simulink model "TST_StSys_StrtCtl"  (R2016b)
settings: Solver=FixedStepDiscrete  StartTime=0.0  StopTime=simTime  FixedStep=sampleTime  RelTol=1e-3
values from neighbouring files (symbols this model uses):
  testCase = 1    [initTST_StSys_StrtCtl_001.m]    (also in initTST_StSys_StrtCtl_002.m = 2)
libraries: simulink x5, UnitTest_Lib x2
settings Model: Creator=xuxingpei  LastModifiedBy=xuxingpei
settings DebuggingCC: SignalRangeChecking=error

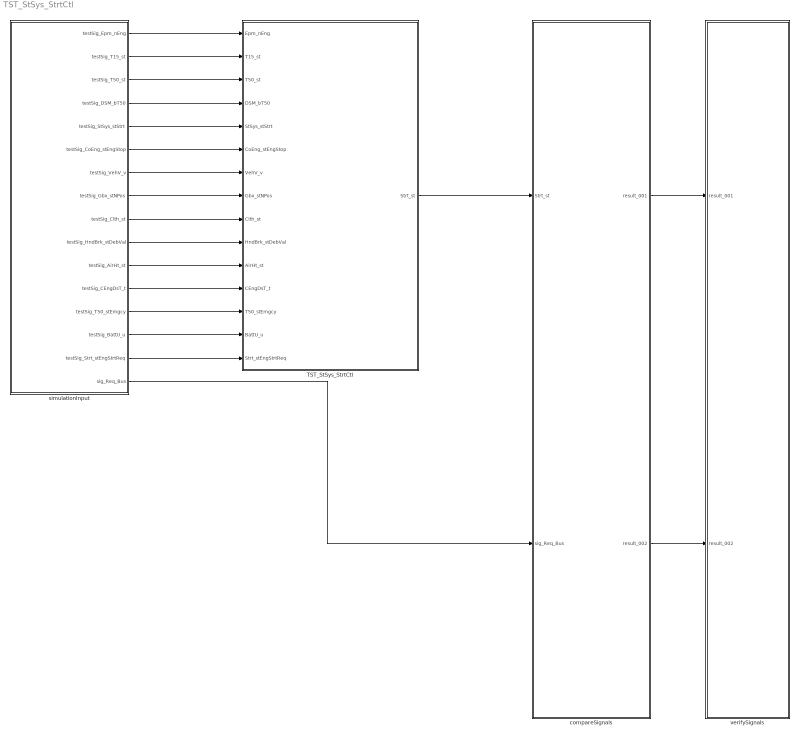
== system TST_StSys_StrtCtl ==
  TST_StSys_StrtCtl : Subsystem
  compareSignals : Subsystem
  simulationInput : Subsystem
  verifySignals : Subsystem
  wires:
  simulationInput/1(testSig_Epm_nEng) -> TST_StSys_StrtCtl/1(Epm_nEng)
  simulationInput/2(testSig_T15_st) -> TST_StSys_StrtCtl/2(T15_st)
  simulationInput/3(testSig_T50_st) -> TST_StSys_StrtCtl/3(T50_st)
  simulationInput/4(testSig_DSM_bT50) -> TST_StSys_StrtCtl/4(DSM_bT50)
  simulationInput/5(testSig_StSys_stStrt) -> TST_StSys_StrtCtl/5(StSys_stStrt)
  simulationInput/6(testSig_CoEng_stEngStop) -> TST_StSys_StrtCtl/6(CoEng_stEngStop)
  simulationInput/7(testSig_VehV_v) -> TST_StSys_StrtCtl/7(VehV_v)
  simulationInput/8(testSig_Gbx_stNPos) -> TST_StSys_StrtCtl/8(Gbx_stNPos)
  simulationInput/9(testSig_Clth_st) -> TST_StSys_StrtCtl/9(Clth_st)
  simulationInput/10(testSig_HndBrk_stDebVal) -> TST_StSys_StrtCtl/10(HndBrk_stDebVal)
  simulationInput/11(testSig_AirHt_st) -> TST_StSys_StrtCtl/11(AirHt_st)
  simulationInput/12(testSig_CEngDsT_t) -> TST_StSys_StrtCtl/12(CEngDsT_t)
  simulationInput/13(testSig_T50_stEmgcy) -> TST_StSys_StrtCtl/13(T50_stEmgcy)
  simulationInput/14(testSig_BattU_u) -> TST_StSys_StrtCtl/14(BattU_u)
  simulationInput/15(testSig_Strt_stEngStrtReq) -> TST_StSys_StrtCtl/15(Strt_stEngStrtReq)
  TST_StSys_StrtCtl/1(Strt_st) -> compareSignals/1(Strt_st)
  simulationInput/16(sig_Req_Bus) -> compareSignals/2(sig_Req_Bus)
  compareSignals/1(result_001) -> verifySignals/1(result_001)
  compareSignals/2(result_002) -> verifySignals/2(result_002)

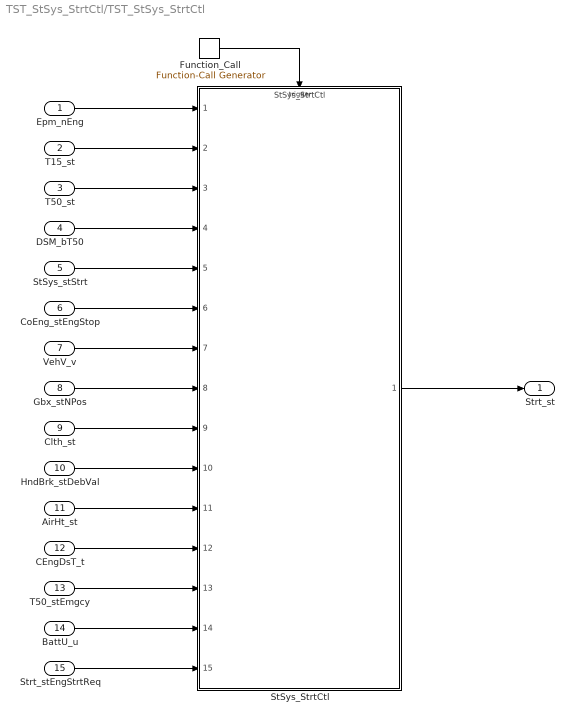
== system TST_StSys_StrtCtl/TST_StSys_StrtCtl ==
  Epm_nEng : Inport
  T15_st : Inport  Port=2
  T50_st : Inport  Port=3
  DSM_bT50 : Inport  Port=4
  StSys_stStrt : Inport  Port=5
  CoEng_stEngStop : Inport  Port=6
  VehV_v : Inport  Port=7
  Gbx_stNPos : Inport  Port=8
  Clth_st : Inport  Port=9
  HndBrk_stDebVal : Inport  Port=10
  AirHt_st : Inport  Port=11
  CEngDsT_t : Inport  Port=12
  T50_stEmgcy : Inport  Port=13
  BattU_u : Inport  Port=14
  Strt_stEngStrtReq : Inport  Port=15
  Function_Call : simulink/Ports & Subsystems/Function-Call Generator  sample_time=sampleTime  numberOfIterations=1
  StSys_StrtCtl : ModelReference  ModelNameDialog=StSys_StrtCtl  SimulationMode=Normal  ModelReferenceVersion=1.583  TriggerPortName=function  TriggerPortTriggerType=function-call  TriggerPortStatesWhenEnabling=held
  Strt_st : Outport
  wires:
  Function_Call/1 -> StSys_StrtCtl/Trigger
  Epm_nEng/1 -> StSys_StrtCtl/1
  T15_st/1 -> StSys_StrtCtl/2
  T50_st/1 -> StSys_StrtCtl/3
  DSM_bT50/1 -> StSys_StrtCtl/4
  StSys_stStrt/1 -> StSys_StrtCtl/5
  CoEng_stEngStop/1 -> StSys_StrtCtl/6
  VehV_v/1 -> StSys_StrtCtl/7
  Gbx_stNPos/1 -> StSys_StrtCtl/8
  Clth_st/1 -> StSys_StrtCtl/9
  HndBrk_stDebVal/1 -> StSys_StrtCtl/10
  AirHt_st/1 -> StSys_StrtCtl/11
  CEngDsT_t/1 -> StSys_StrtCtl/12
  T50_stEmgcy/1 -> StSys_StrtCtl/13
  BattU_u/1 -> StSys_StrtCtl/14
  Strt_stEngStrtReq/1 -> StSys_StrtCtl/15
  StSys_StrtCtl/1 -> Strt_st/1

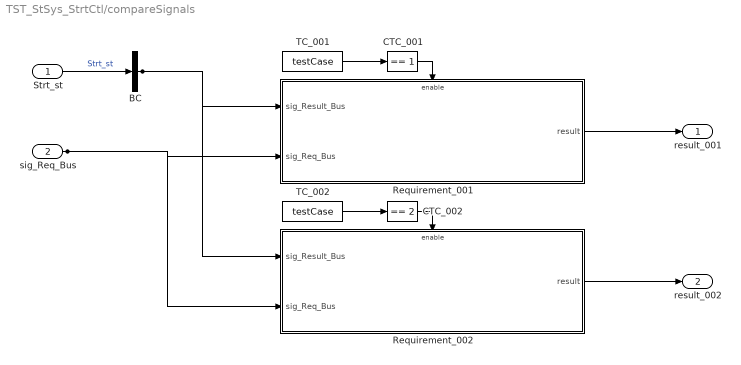
== system TST_StSys_StrtCtl/compareSignals ==
  Strt_st : Inport
  sig_Req_Bus : Inport  Port=2
  BC : BusCreator  Inputs=1
  CTC_001 : simulink/Logic and Bit Operations/Compare To Constant  relop===  const=1  OutDataTypeStr=boolean
  CTC_002 : simulink/Logic and Bit Operations/Compare To Constant  relop===  const=2  OutDataTypeStr=boolean
  Requirement_001 : Subsystem
  Requirement_002 : Subsystem
  TC_001 : Constant  Value=testCase
  TC_002 : Constant  Value=testCase
  result_001 : Outport
  result_002 : Outport  Port=2
  wires:
  Strt_st/1 -> BC/1  "Strt_st"
  TC_001/1 -> CTC_001/1
  CTC_001/1 -> Requirement_001/Enable
  sig_Req_Bus/1 -> Requirement_001/2(sig_Req_Bus), Requirement_002/2(sig_Req_Bus)
  BC/1 -> Requirement_001/1(sig_Result_Bus), Requirement_002/1(sig_Result_Bus)
  Requirement_001/1(result) -> result_001/1
  TC_002/1 -> CTC_002/1
  CTC_002/1 -> Requirement_002/Enable
  Requirement_002/1(result) -> result_002/1

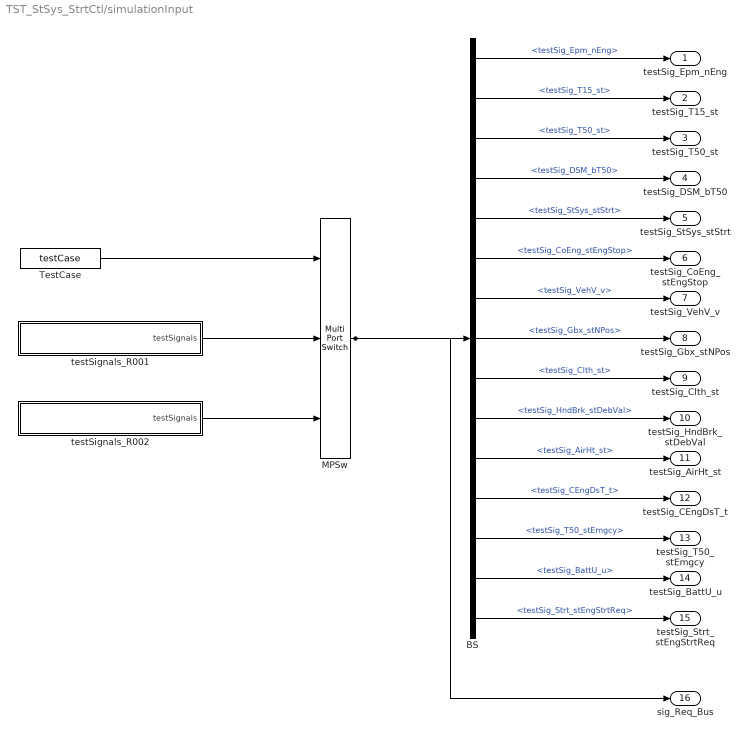
== system TST_StSys_StrtCtl/simulationInput ==
  BS : BusSelector  OutputSignals=testSig_Epm_nEng,testSig_T15_st,testSig_T50_st,testSig_DSM_bT50,testSig_StSys_stStrt,testSig_CoEng_stEngStop,testSig_VehV_v,testSig_Gbx_stNPos,testSig_Clth_st,testSig_HndBrk_stDebVal,testSig_AirHt_st,testSig_CEngDsT_t,testSig_T50_stEmgcy,testSig_BattU_u,testSig_Strt_stEngStrtReq
  MPSw : MultiPortSwitch  Inputs=2  SaturateOnIntegerOverflow=on  InputSameDT=on
  TestCase : Constant  Value=testCase
  testSignals_R001 : Subsystem
  testSignals_R002 : Subsystem
  testSig_Epm_nEng : Outport
  testSig_T15_st : Outport  Port=2
  testSig_T50_st : Outport  Port=3
  testSig_DSM_bT50 : Outport  Port=4
  testSig_StSys_stStrt : Outport  Port=5
  testSig_CoEng_stEngStop : Outport  Port=6
  testSig_VehV_v : Outport  Port=7
  testSig_Gbx_stNPos : Outport  Port=8
  testSig_Clth_st : Outport  Port=9
  testSig_HndBrk_stDebVal : Outport  Port=10
  testSig_AirHt_st : Outport  Port=11
  testSig_CEngDsT_t : Outport  Port=12
  testSig_T50_stEmgcy : Outport  Port=13
  testSig_BattU_u : Outport  Port=14
  testSig_Strt_stEngStrtReq : Outport  Port=15
  sig_Req_Bus : Outport  Port=16
  wires:
  BS/1 -> testSig_Epm_nEng/1  "<testSig_Epm_nEng>"
  BS/2 -> testSig_T15_st/1  "<testSig_T15_st>"
  BS/3 -> testSig_T50_st/1  "<testSig_T50_st>"
  BS/4 -> testSig_DSM_bT50/1  "<testSig_DSM_bT50>"
  BS/5 -> testSig_StSys_stStrt/1  "<testSig_StSys_stStrt>"
  BS/6 -> testSig_CoEng_stEngStop/1  "<testSig_CoEng_stEngStop>"
  BS/7 -> testSig_VehV_v/1  "<testSig_VehV_v>"
  BS/8 -> testSig_Gbx_stNPos/1  "<testSig_Gbx_stNPos>"
  BS/9 -> testSig_Clth_st/1  "<testSig_Clth_st>"
  BS/10 -> testSig_HndBrk_stDebVal/1  "<testSig_HndBrk_stDebVal>"
  BS/11 -> testSig_AirHt_st/1  "<testSig_AirHt_st>"
  BS/12 -> testSig_CEngDsT_t/1  "<testSig_CEngDsT_t>"
  BS/13 -> testSig_T50_stEmgcy/1  "<testSig_T50_stEmgcy>"
  BS/14 -> testSig_BattU_u/1  "<testSig_BattU_u>"
  BS/15 -> testSig_Strt_stEngStrtReq/1  "<testSig_Strt_stEngStrtReq>"
  MPSw/1 -> BS/1, sig_Req_Bus/1
  TestCase/1 -> MPSw/1
  testSignals_R001/1(testSignals) -> MPSw/2
  testSignals_R002/1(testSignals) -> MPSw/3

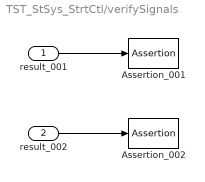
== system TST_StSys_StrtCtl/verifySignals ==
  result_001 : Inport
  result_002 : Inport  Port=2
  Assertion_001 : Assertion  Enabled=off
  Assertion_002 : Assertion  Enabled=off
  wires:
  result_001/1 -> Assertion_001/1
  result_002/1 -> Assertion_002/1

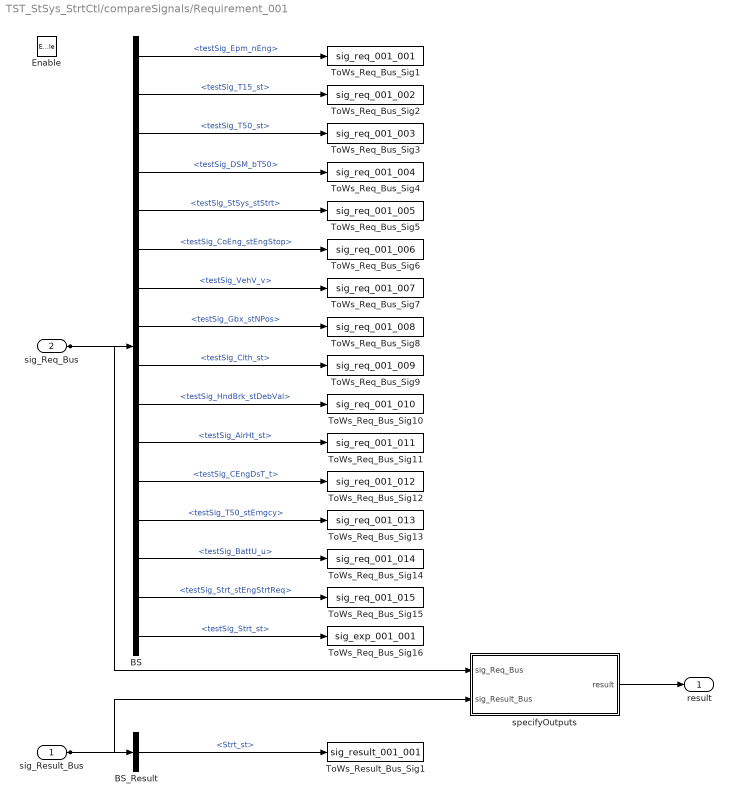
== system TST_StSys_StrtCtl/compareSignals/Requirement_001 ==
  sig_Result_Bus : Inport
  sig_Req_Bus : Inport  Port=2
  Enable : EnablePort
  BS : BusSelector  OutputSignals=testSig_Epm_nEng,testSig_T15_st,testSig_T50_st,testSig_DSM_bT50,testSig_StSys_stStrt,testSig_CoEng_stEngStop,testSig_VehV_v,testSig_Gbx_stNPos,testSig_Clth_st,testSig_HndBrk_stDebVal,testSig_AirHt_st,testSig_CEngDsT_t,testSig_T50_stEmgcy,testSig_BattU_u,testSig_Strt_stEngStrtReq,testSig_Strt_st
  BS_Result : BusSelector  OutputSignals=Strt_st
  ToWs_Req_Bus_Sig1 : ToWorkspace  VariableName=sig_req_001_001  SaveFormat=Structure With Time
  ToWs_Req_Bus_Sig10 : ToWorkspace  VariableName=sig_req_001_010  SaveFormat=Structure With Time
  ToWs_Req_Bus_Sig11 : ToWorkspace  VariableName=sig_req_001_011  SaveFormat=Structure With Time
  ToWs_Req_Bus_Sig12 : ToWorkspace  VariableName=sig_req_001_012  SaveFormat=Structure With Time
  ToWs_Req_Bus_Sig13 : ToWorkspace  VariableName=sig_req_001_013  SaveFormat=Structure With Time
  ToWs_Req_Bus_Sig14 : ToWorkspace  VariableName=sig_req_001_014  SaveFormat=Structure With Time
  ToWs_Req_Bus_Sig15 : ToWorkspace  VariableName=sig_req_001_015  SaveFormat=Structure With Time
  ToWs_Req_Bus_Sig16 : ToWorkspace  VariableName=sig_exp_001_001  SaveFormat=Structure With Time
  ToWs_Req_Bus_Sig2 : ToWorkspace  VariableName=sig_req_001_002  SaveFormat=Structure With Time
  ToWs_Req_Bus_Sig3 : ToWorkspace  VariableName=sig_req_001_003  SaveFormat=Structure With Time
  ToWs_Req_Bus_Sig4 : ToWorkspace  VariableName=sig_req_001_004  SaveFormat=Structure With Time
  ToWs_Req_Bus_Sig5 : ToWorkspace  VariableName=sig_req_001_005  SaveFormat=Structure With Time
  ToWs_Req_Bus_Sig6 : ToWorkspace  VariableName=sig_req_001_006  SaveFormat=Structure With Time
  ToWs_Req_Bus_Sig7 : ToWorkspace  VariableName=sig_req_001_007  SaveFormat=Structure With Time
  ToWs_Req_Bus_Sig8 : ToWorkspace  VariableName=sig_req_001_008  SaveFormat=Structure With Time
  ToWs_Req_Bus_Sig9 : ToWorkspace  VariableName=sig_req_001_009  SaveFormat=Structure With Time
  ToWs_Result_Bus_Sig1 : ToWorkspace  VariableName=sig_result_001_001  SaveFormat=Structure With Time
  specifyOutputs : Subsystem
  result : Outport
  wires:
  sig_Req_Bus/1 -> BS/1, specifyOutputs/1(sig_Req_Bus)
  BS/1 -> ToWs_Req_Bus_Sig1/1  "<testSig_Epm_nEng>"
  BS/2 -> ToWs_Req_Bus_Sig2/1  "<testSig_T15_st>"
  BS/3 -> ToWs_Req_Bus_Sig3/1  "<testSig_T50_st>"
  BS/4 -> ToWs_Req_Bus_Sig4/1  "<testSig_DSM_bT50>"
  BS/5 -> ToWs_Req_Bus_Sig5/1  "<testSig_StSys_stStrt>"
  BS/6 -> ToWs_Req_Bus_Sig6/1  "<testSig_CoEng_stEngStop>"
  BS/7 -> ToWs_Req_Bus_Sig7/1  "<testSig_VehV_v>"
  BS/8 -> ToWs_Req_Bus_Sig8/1  "<testSig_Gbx_stNPos>"
  BS/9 -> ToWs_Req_Bus_Sig9/1  "<testSig_Clth_st>"
  BS/10 -> ToWs_Req_Bus_Sig10/1  "<testSig_HndBrk_stDebVal>"
  BS/11 -> ToWs_Req_Bus_Sig11/1  "<testSig_AirHt_st>"
  BS/12 -> ToWs_Req_Bus_Sig12/1  "<testSig_CEngDsT_t>"
  BS/13 -> ToWs_Req_Bus_Sig13/1  "<testSig_T50_stEmgcy>"
  BS/14 -> ToWs_Req_Bus_Sig14/1  "<testSig_BattU_u>"
  BS/15 -> ToWs_Req_Bus_Sig15/1  "<testSig_Strt_stEngStrtReq>"
  BS/16 -> ToWs_Req_Bus_Sig16/1  "<testSig_Strt_st>"
  sig_Result_Bus/1 -> BS_Result/1, specifyOutputs/2(sig_Result_Bus)
  BS_Result/1 -> ToWs_Result_Bus_Sig1/1  "<Strt_st>"
  specifyOutputs/1(result) -> result/1

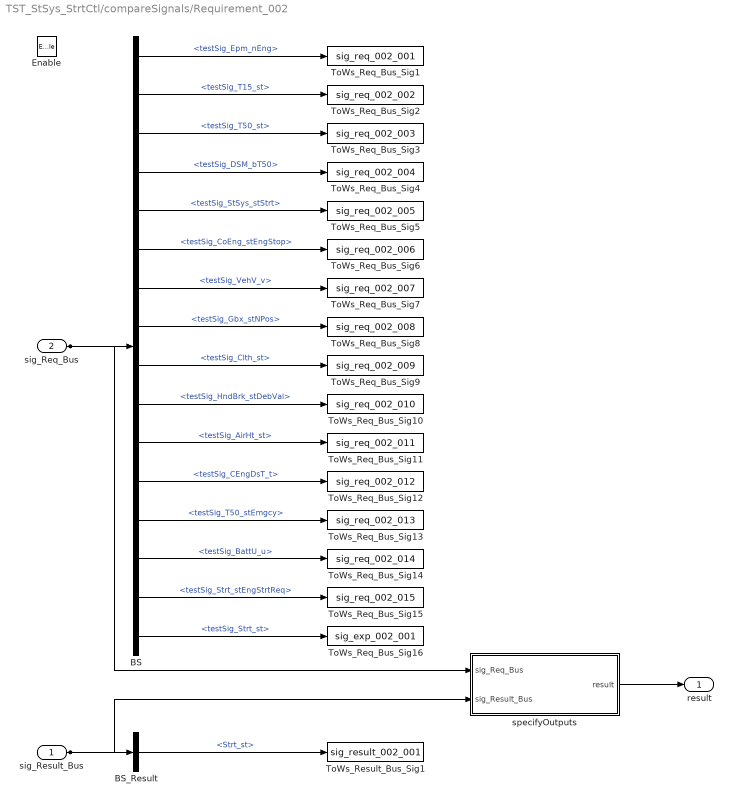
== system TST_StSys_StrtCtl/compareSignals/Requirement_002 ==
  sig_Result_Bus : Inport
  sig_Req_Bus : Inport  Port=2
  Enable : EnablePort
  BS : BusSelector  OutputSignals=testSig_Epm_nEng,testSig_T15_st,testSig_T50_st,testSig_DSM_bT50,testSig_StSys_stStrt,testSig_CoEng_stEngStop,testSig_VehV_v,testSig_Gbx_stNPos,testSig_Clth_st,testSig_HndBrk_stDebVal,testSig_AirHt_st,testSig_CEngDsT_t,testSig_T50_stEmgcy,testSig_BattU_u,testSig_Strt_stEngStrtReq,testSig_Strt_st
  BS_Result : BusSelector  OutputSignals=Strt_st
  ToWs_Req_Bus_Sig1 : ToWorkspace  VariableName=sig_req_002_001  SaveFormat=Structure With Time
  ToWs_Req_Bus_Sig10 : ToWorkspace  VariableName=sig_req_002_010  SaveFormat=Structure With Time
  ToWs_Req_Bus_Sig11 : ToWorkspace  VariableName=sig_req_002_011  SaveFormat=Structure With Time
  ToWs_Req_Bus_Sig12 : ToWorkspace  VariableName=sig_req_002_012  SaveFormat=Structure With Time
  ToWs_Req_Bus_Sig13 : ToWorkspace  VariableName=sig_req_002_013  SaveFormat=Structure With Time
  ToWs_Req_Bus_Sig14 : ToWorkspace  VariableName=sig_req_002_014  SaveFormat=Structure With Time
  ToWs_Req_Bus_Sig15 : ToWorkspace  VariableName=sig_req_002_015  SaveFormat=Structure With Time
  ToWs_Req_Bus_Sig16 : ToWorkspace  VariableName=sig_exp_002_001  SaveFormat=Structure With Time
  ToWs_Req_Bus_Sig2 : ToWorkspace  VariableName=sig_req_002_002  SaveFormat=Structure With Time
  ToWs_Req_Bus_Sig3 : ToWorkspace  VariableName=sig_req_002_003  SaveFormat=Structure With Time
  ToWs_Req_Bus_Sig4 : ToWorkspace  VariableName=sig_req_002_004  SaveFormat=Structure With Time
  ToWs_Req_Bus_Sig5 : ToWorkspace  VariableName=sig_req_002_005  SaveFormat=Structure With Time
  ToWs_Req_Bus_Sig6 : ToWorkspace  VariableName=sig_req_002_006  SaveFormat=Structure With Time
  ToWs_Req_Bus_Sig7 : ToWorkspace  VariableName=sig_req_002_007  SaveFormat=Structure With Time
  ToWs_Req_Bus_Sig8 : ToWorkspace  VariableName=sig_req_002_008  SaveFormat=Structure With Time
  ToWs_Req_Bus_Sig9 : ToWorkspace  VariableName=sig_req_002_009  SaveFormat=Structure With Time
  ToWs_Result_Bus_Sig1 : ToWorkspace  VariableName=sig_result_002_001  SaveFormat=Structure With Time
  specifyOutputs : Subsystem
  result : Outport
  wires:
  sig_Req_Bus/1 -> BS/1, specifyOutputs/1(sig_Req_Bus)
  BS/1 -> ToWs_Req_Bus_Sig1/1  "<testSig_Epm_nEng>"
  BS/2 -> ToWs_Req_Bus_Sig2/1  "<testSig_T15_st>"
  BS/3 -> ToWs_Req_Bus_Sig3/1  "<testSig_T50_st>"
  BS/4 -> ToWs_Req_Bus_Sig4/1  "<testSig_DSM_bT50>"
  BS/5 -> ToWs_Req_Bus_Sig5/1  "<testSig_StSys_stStrt>"
  BS/6 -> ToWs_Req_Bus_Sig6/1  "<testSig_CoEng_stEngStop>"
  BS/7 -> ToWs_Req_Bus_Sig7/1  "<testSig_VehV_v>"
  BS/8 -> ToWs_Req_Bus_Sig8/1  "<testSig_Gbx_stNPos>"
  BS/9 -> ToWs_Req_Bus_Sig9/1  "<testSig_Clth_st>"
  BS/10 -> ToWs_Req_Bus_Sig10/1  "<testSig_HndBrk_stDebVal>"
  BS/11 -> ToWs_Req_Bus_Sig11/1  "<testSig_AirHt_st>"
  BS/12 -> ToWs_Req_Bus_Sig12/1  "<testSig_CEngDsT_t>"
  BS/13 -> ToWs_Req_Bus_Sig13/1  "<testSig_T50_stEmgcy>"
  BS/14 -> ToWs_Req_Bus_Sig14/1  "<testSig_BattU_u>"
  BS/15 -> ToWs_Req_Bus_Sig15/1  "<testSig_Strt_stEngStrtReq>"
  BS/16 -> ToWs_Req_Bus_Sig16/1  "<testSig_Strt_st>"
  sig_Result_Bus/1 -> BS_Result/1, specifyOutputs/2(sig_Result_Bus)
  BS_Result/1 -> ToWs_Result_Bus_Sig1/1  "<Strt_st>"
  specifyOutputs/1(result) -> result/1

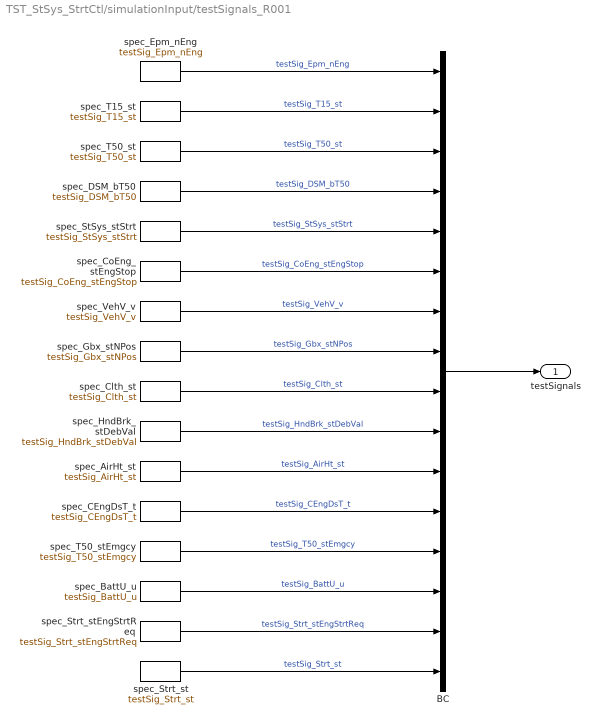
== system TST_StSys_StrtCtl/simulationInput/testSignals_R001 ==
  BC : BusCreator  Inputs=16
  spec_AirHt_st : FromWorkspace  VariableName=testSig_AirHt_st  Interpolate=off  OutputAfterFinalValue=Holding final value
  spec_BattU_u : FromWorkspace  VariableName=testSig_BattU_u  Interpolate=off  OutputAfterFinalValue=Holding final value
  spec_CEngDsT_t : FromWorkspace  VariableName=testSig_CEngDsT_t  Interpolate=off  OutputAfterFinalValue=Holding final value
  spec_Clth_st : FromWorkspace  VariableName=testSig_Clth_st  Interpolate=off  OutputAfterFinalValue=Holding final value
  spec_CoEng_stEngStop : FromWorkspace  VariableName=testSig_CoEng_stEngStop  Interpolate=off  OutputAfterFinalValue=Holding final value
  spec_DSM_bT50 : FromWorkspace  VariableName=testSig_DSM_bT50  Interpolate=off  OutputAfterFinalValue=Holding final value
  spec_Epm_nEng : FromWorkspace  VariableName=testSig_Epm_nEng  Interpolate=off  OutputAfterFinalValue=Holding final value
  spec_Gbx_stNPos : FromWorkspace  VariableName=testSig_Gbx_stNPos  Interpolate=off  OutputAfterFinalValue=Holding final value
  spec_HndBrk_stDebVal : FromWorkspace  VariableName=testSig_HndBrk_stDebVal  Interpolate=off  OutputAfterFinalValue=Holding final value
  spec_StSys_stStrt : FromWorkspace  VariableName=testSig_StSys_stStrt  Interpolate=off  OutputAfterFinalValue=Holding final value
  spec_Strt_st : FromWorkspace  VariableName=testSig_Strt_st  Interpolate=off  OutputAfterFinalValue=Holding final value
  spec_Strt_stEngStrtReq : FromWorkspace  VariableName=testSig_Strt_stEngStrtReq  Interpolate=off  OutputAfterFinalValue=Holding final value
  spec_T15_st : FromWorkspace  VariableName=testSig_T15_st  Interpolate=off  OutputAfterFinalValue=Holding final value
  spec_T50_st : FromWorkspace  VariableName=testSig_T50_st  Interpolate=off  OutputAfterFinalValue=Holding final value
  spec_T50_stEmgcy : FromWorkspace  VariableName=testSig_T50_stEmgcy  Interpolate=off  OutputAfterFinalValue=Holding final value
  spec_VehV_v : FromWorkspace  VariableName=testSig_VehV_v  Interpolate=off  OutputAfterFinalValue=Holding final value
  testSignals : Outport
  wires:
  BC/1 -> testSignals/1
  spec_Epm_nEng/1 -> BC/1  "testSig_Epm_nEng"
  spec_T15_st/1 -> BC/2  "testSig_T15_st"
  spec_T50_st/1 -> BC/3  "testSig_T50_st"
  spec_DSM_bT50/1 -> BC/4  "testSig_DSM_bT50"
  spec_StSys_stStrt/1 -> BC/5  "testSig_StSys_stStrt"
  spec_CoEng_stEngStop/1 -> BC/6  "testSig_CoEng_stEngStop"
  spec_VehV_v/1 -> BC/7  "testSig_VehV_v"
  spec_Gbx_stNPos/1 -> BC/8  "testSig_Gbx_stNPos"
  spec_Clth_st/1 -> BC/9  "testSig_Clth_st"
  spec_HndBrk_stDebVal/1 -> BC/10  "testSig_HndBrk_stDebVal"
  spec_AirHt_st/1 -> BC/11  "testSig_AirHt_st"
  spec_CEngDsT_t/1 -> BC/12  "testSig_CEngDsT_t"
  spec_T50_stEmgcy/1 -> BC/13  "testSig_T50_stEmgcy"
  spec_BattU_u/1 -> BC/14  "testSig_BattU_u"
  spec_Strt_stEngStrtReq/1 -> BC/15  "testSig_Strt_stEngStrtReq"
  spec_Strt_st/1 -> BC/16  "testSig_Strt_st"

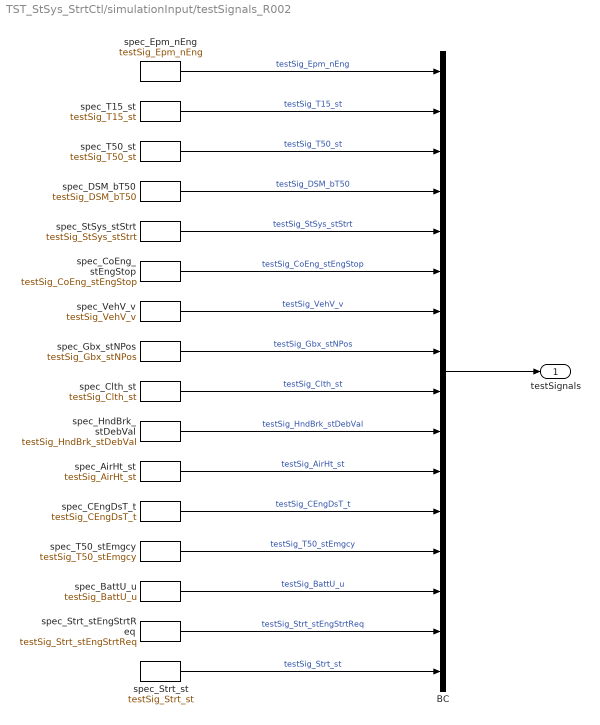
== system TST_StSys_StrtCtl/simulationInput/testSignals_R002 ==
  BC : BusCreator  Inputs=16
  spec_AirHt_st : FromWorkspace  VariableName=testSig_AirHt_st  Interpolate=off  OutputAfterFinalValue=Holding final value
  spec_BattU_u : FromWorkspace  VariableName=testSig_BattU_u  Interpolate=off  OutputAfterFinalValue=Holding final value
  spec_CEngDsT_t : FromWorkspace  VariableName=testSig_CEngDsT_t  Interpolate=off  OutputAfterFinalValue=Holding final value
  spec_Clth_st : FromWorkspace  VariableName=testSig_Clth_st  Interpolate=off  OutputAfterFinalValue=Holding final value
  spec_CoEng_stEngStop : FromWorkspace  VariableName=testSig_CoEng_stEngStop  Interpolate=off  OutputAfterFinalValue=Holding final value
  spec_DSM_bT50 : FromWorkspace  VariableName=testSig_DSM_bT50  Interpolate=off  OutputAfterFinalValue=Holding final value
  spec_Epm_nEng : FromWorkspace  VariableName=testSig_Epm_nEng  Interpolate=off  OutputAfterFinalValue=Holding final value
  spec_Gbx_stNPos : FromWorkspace  VariableName=testSig_Gbx_stNPos  Interpolate=off  OutputAfterFinalValue=Holding final value
  spec_HndBrk_stDebVal : FromWorkspace  VariableName=testSig_HndBrk_stDebVal  Interpolate=off  OutputAfterFinalValue=Holding final value
  spec_StSys_stStrt : FromWorkspace  VariableName=testSig_StSys_stStrt  Interpolate=off  OutputAfterFinalValue=Holding final value
  spec_Strt_st : FromWorkspace  VariableName=testSig_Strt_st  Interpolate=off  OutputAfterFinalValue=Holding final value
  spec_Strt_stEngStrtReq : FromWorkspace  VariableName=testSig_Strt_stEngStrtReq  Interpolate=off  OutputAfterFinalValue=Holding final value
  spec_T15_st : FromWorkspace  VariableName=testSig_T15_st  Interpolate=off  OutputAfterFinalValue=Holding final value
  spec_T50_st : FromWorkspace  VariableName=testSig_T50_st  Interpolate=off  OutputAfterFinalValue=Holding final value
  spec_T50_stEmgcy : FromWorkspace  VariableName=testSig_T50_stEmgcy  Interpolate=off  OutputAfterFinalValue=Holding final value
  spec_VehV_v : FromWorkspace  VariableName=testSig_VehV_v  Interpolate=off  OutputAfterFinalValue=Holding final value
  testSignals : Outport
  wires:
  BC/1 -> testSignals/1
  spec_Epm_nEng/1 -> BC/1  "testSig_Epm_nEng"
  spec_T15_st/1 -> BC/2  "testSig_T15_st"
  spec_T50_st/1 -> BC/3  "testSig_T50_st"
  spec_DSM_bT50/1 -> BC/4  "testSig_DSM_bT50"
  spec_StSys_stStrt/1 -> BC/5  "testSig_StSys_stStrt"
  spec_CoEng_stEngStop/1 -> BC/6  "testSig_CoEng_stEngStop"
  spec_VehV_v/1 -> BC/7  "testSig_VehV_v"
  spec_Gbx_stNPos/1 -> BC/8  "testSig_Gbx_stNPos"
  spec_Clth_st/1 -> BC/9  "testSig_Clth_st"
  spec_HndBrk_stDebVal/1 -> BC/10  "testSig_HndBrk_stDebVal"
  spec_AirHt_st/1 -> BC/11  "testSig_AirHt_st"
  spec_CEngDsT_t/1 -> BC/12  "testSig_CEngDsT_t"
  spec_T50_stEmgcy/1 -> BC/13  "testSig_T50_stEmgcy"
  spec_BattU_u/1 -> BC/14  "testSig_BattU_u"
  spec_Strt_stEngStrtReq/1 -> BC/15  "testSig_Strt_stEngStrtReq"
  spec_Strt_st/1 -> BC/16  "testSig_Strt_st"

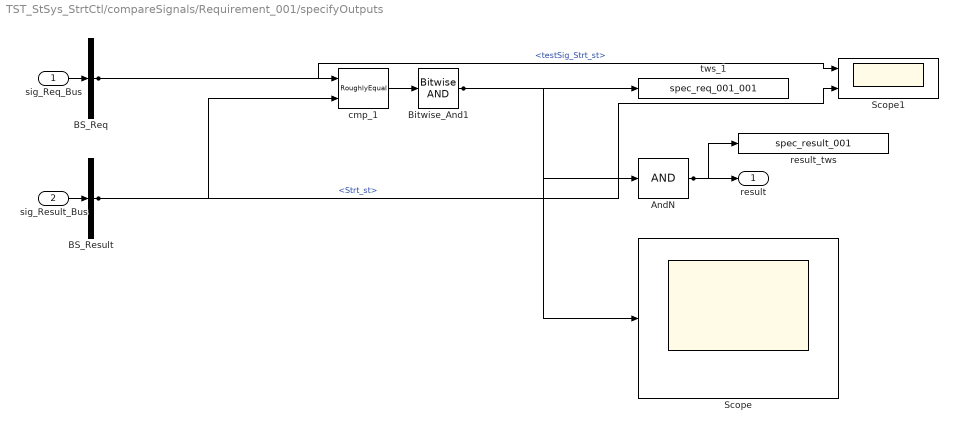
== system TST_StSys_StrtCtl/compareSignals/Requirement_001/specifyOutputs ==
  sig_Req_Bus : Inport
  sig_Result_Bus : Inport  Port=2
  AndN : Logic  Inputs=1
  BS_Req : BusSelector  OutputSignals=testSig_Strt_st
  BS_Result : BusSelector  OutputSignals=Strt_st
  Bitwise_And1 : simulink/Logic and Bit Operations/Bitwise Operator  logicop=AND  UseBitMask=off  BitMask=bin2dec('11011001')  BitMaskRealWorld=Stored Integer
  Scope : Scope
  Scope1 : Scope  NumInputPorts=2
  cmp_1 : UnitTest_Lib/RoughlyEqual  slope=0.1
  result_tws : ToWorkspace  VariableName=spec_result_001
  tws_1 : ToWorkspace  VariableName=spec_req_001_001
  result : Outport
  wires:
  sig_Req_Bus/1 -> BS_Req/1
  sig_Result_Bus/1 -> BS_Result/1
  AndN/1 -> result/1, result_tws/1
  BS_Req/1 -> cmp_1/1, Scope1/1  "<testSig_Strt_st>"
  BS_Result/1 -> cmp_1/2, Scope1/2  "<Strt_st>"
  cmp_1/1 -> Bitwise_And1/1
  Bitwise_And1/1 -> tws_1/1, AndN/1, Scope/1

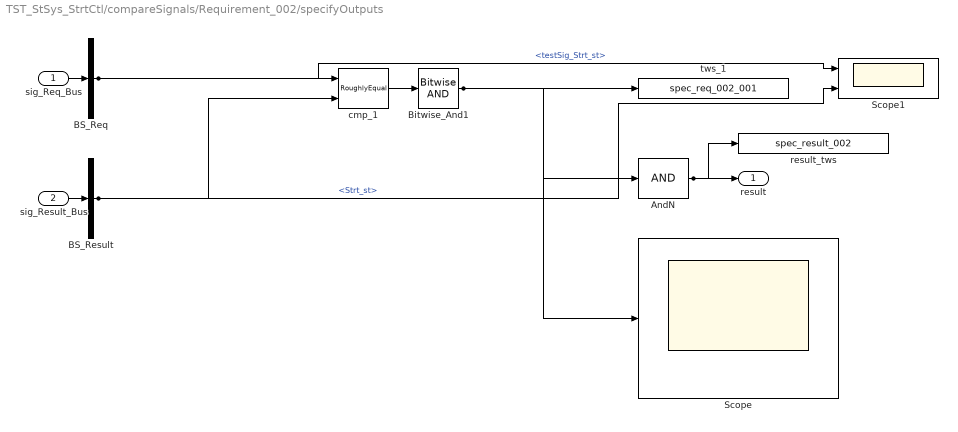
== system TST_StSys_StrtCtl/compareSignals/Requirement_002/specifyOutputs ==
  sig_Req_Bus : Inport
  sig_Result_Bus : Inport  Port=2
  AndN : Logic  Inputs=1
  BS_Req : BusSelector  OutputSignals=testSig_Strt_st
  BS_Result : BusSelector  OutputSignals=Strt_st
  Bitwise_And1 : simulink/Logic and Bit Operations/Bitwise Operator  logicop=AND  UseBitMask=off  BitMask=bin2dec('11011001')  BitMaskRealWorld=Stored Integer
  Scope : Scope
  Scope1 : Scope  NumInputPorts=2
  cmp_1 : UnitTest_Lib/RoughlyEqual  slope=0.1
  result_tws : ToWorkspace  VariableName=spec_result_002
  tws_1 : ToWorkspace  VariableName=spec_req_002_001
  result : Outport
  wires:
  sig_Req_Bus/1 -> BS_Req/1
  sig_Result_Bus/1 -> BS_Result/1
  AndN/1 -> result/1, result_tws/1
  BS_Req/1 -> cmp_1/1, Scope1/1  "<testSig_Strt_st>"
  BS_Result/1 -> cmp_1/2, Scope1/2  "<Strt_st>"
  cmp_1/1 -> Bitwise_And1/1
  Bitwise_And1/1 -> tws_1/1, AndN/1, Scope/1
